simulink model "Sim03_TrackingDiff_DT"  (R2020a)
settings: Solver=FixedStepAuto  StartTime=0.0  StopTime=T  FixedStep=Ts  RelTol=1e-3
values from neighbouring files (symbols this model uses):
  A = 1    [Sim02_Differentiator.m]    (also in Sim03_Differentiator.m)
  h = 10*Ts    (= 0.001)    [Sim03_Differentiator.m]
  omg = 1    [Sim02_Differentiator.m]    (also in Sim03_Differentiator.m = 2*pi*f(k))
  r = 20    [Sim03_Differentiator.m]
  Ts = 1e-3    (= 0.001)    [Sim01_Stability.m]    (also in Sim02_Differentiator.m = 1e-05; Sim03_Differentiator.m = 0.0001)
  xn = 0.1    [Sim02_Differentiator.m]    (also in Sim03_Differentiator.m)
  xnFlag = 1    [Sim02_Differentiator.m]    (also in Sim03_Differentiator.m = 0)
libraries: simulink x1
settings Model: Creator=XiaoCY  LastModifiedBy=XiaoCY
settings DataIOCC: ReturnWorkspaceOutputs=off

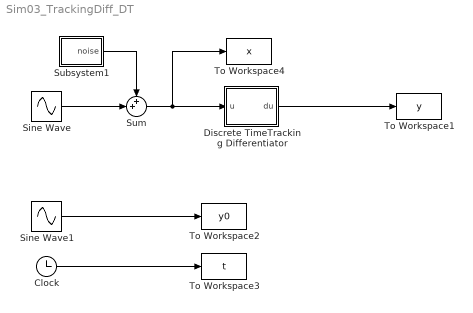
== system Sim03_TrackingDiff_DT ==
  Clock : Clock
  Discrete TimeTracking Differentiator : Subsystem  mask{r=r, h=h, Ts=Ts}
      mask prompts: r "Rate factor"; h "Step time"; Ts "Sample time"
      mask Display: disp('TD')
  Sine Wave : Sin  Amplitude=A  Frequency=omg  SampleTime=0
  Sine Wave1 : Sin  Amplitude=A  Frequency=omg  Phase=pi/2  SampleTime=0
  Subsystem1 : Subsystem
  Sum : Sum  Inputs=++|
  To Workspace1 : ToWorkspace  VariableName=y  SampleTime=Ts
  To Workspace2 : ToWorkspace  VariableName=y0  SampleTime=Ts
  To Workspace3 : ToWorkspace  VariableName=t  SampleTime=Ts
  To Workspace4 : ToWorkspace  VariableName=x  SampleTime=Ts
  wires:
  Clock/1 -> To Workspace3/1
  Sine Wave/1 -> Sum/2
  Sum/1 -> To Workspace4/1, Discrete TimeTracking Differentiator/1(u)
  Discrete TimeTracking Differentiator/1(du) -> To Workspace1/1
  Sine Wave1/1 -> To Workspace2/1
  Subsystem1/1(noise) -> Sum/1

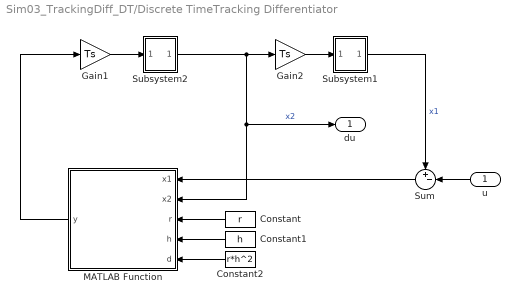
== system Sim03_TrackingDiff_DT/Discrete TimeTracking Differentiator ==
  u : Inport
  Constant : Constant  Value=r
  Constant1 : Constant  Value=h
  Constant2 : Constant  Value=r*h^2
  Gain1 : Gain  Gain=Ts
  Gain2 : Gain  Gain=Ts
  MATLAB Function : MATLAB Function  TreatAsAtomicUnit=on  SystemSampleTime=Ts
  Subsystem1 : Subsystem
      mask Display: disp('\Sigma','interpreter','tex')
  Subsystem2 : Subsystem
      mask Display: disp('\Sigma','interpreter','tex')
  Sum : Sum  Inputs=+-|
  du : Outport
  wires:
  Subsystem2/1(Out1) -> Gain2/1, MATLAB Function/2(x2), du/1  "x2"
  Constant/1 -> MATLAB Function/3(r)
  Constant1/1 -> MATLAB Function/4(h)
  Constant2/1 -> MATLAB Function/5(d)
  Subsystem1/1(Out1) -> Sum/1  "x1"
  MATLAB Function/1(y) -> Gain1/1
  u/1 -> Sum/2
  Sum/1 -> MATLAB Function/1(x1)
  Gain1/1 -> Subsystem2/1(In1)
  Gain2/1 -> Subsystem1/1(In1)

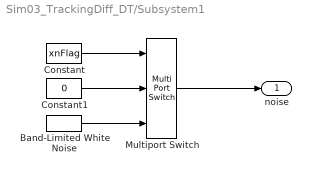
== system Sim03_TrackingDiff_DT/Subsystem1 ==
  Band-Limited White Noise : simulink/Sources/Band-Limited White Noise  Cov=xn^2*Ts  Ts=Ts  seed=[23341]
  Constant : Constant  Value=xnFlag
  Constant1 : Constant  Value=0
  Multiport Switch : MultiPortSwitch  DataPortOrder=Zero-based contiguous  Inputs=2  zeroidx=on
  noise : Outport
  wires:
  Band-Limited White Noise/1 -> Multiport Switch/3
  Constant1/1 -> Multiport Switch/2
  Multiport Switch/1 -> noise/1
  Constant/1 -> Multiport Switch/1

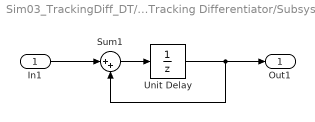
== system Sim03_TrackingDiff_DT/Discrete TimeTracking Differentiator/Subsystem1 ==
  In1 : Inport
  Sum1 : Sum  Inputs=|++
  Unit Delay : UnitDelay  SampleTime=Ts  HasFrameUpgradeWarning=on
  Out1 : Outport
  wires:
  Sum1/1 -> Unit Delay/1
  In1/1 -> Sum1/1
  Unit Delay/1 -> Out1/1, Sum1/2

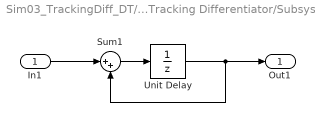
== system Sim03_TrackingDiff_DT/Discrete TimeTracking Differentiator/Subsystem2 ==
  In1 : Inport
  Sum1 : Sum  Inputs=|++
  Unit Delay : UnitDelay  SampleTime=Ts  HasFrameUpgradeWarning=on
  Out1 : Outport
  wires:
  Unit Delay/1 -> Sum1/2, Out1/1
  In1/1 -> Sum1/1
  Sum1/1 -> Unit Delay/1

== matlab function Sim03_TrackingDiff_DT/Discrete TimeTracking Differentiator/MATLAB Function ==
  data: x1 input; y output; x2 input; r input; h input; d input
% Discrete time steepest control synthesis function
% Ref: (ISBN) 978-7-118-05795-9 p.70

%%
function y = fhan(x1,x2,r,h,d)
    fsg = @(x,d) (sign(x+d)-sign(x-d))/2;
    a0 = h*x2;
    y = x1+a0;
    a1 = sqrt(d*(d+8*abs(y)));
    a2 = a0+sign(y)*(a1-d)/2;
    a = (a0+y)*fsg(y,d)+a2*(1-fsg(y,d));
    y = -r*a/d*fsg(a,d)-r*sign(a)*(1-fsg(a,d));
end
